simulink model "test_sim_model_scheduling_v1"  (R2023a)
settings: Solver=VariableStepAuto  StartTime=0.0  StopTime=10.0  RelTol=1e-3
values from neighbouring files (symbols this model uses):
  A = Amatrix(C1, C2, C3, Cf, Cs, Sx, Sy, x0(3), x0(4), w0(1), w0(2), u0(1), epsilon, g, lx, ly, mass, x0(6), x0(5), rho, u0(2), weight_part, wheel_rad)    [model_main_model_scheduling.m]
  A_inv = Amatrix(C1, C2, C3, Cf, Cs, Sx, Sy, x0(3), x0(4), w0_inv(1), w0_inv(2), u0(1), epsilon, g, lx, ly, mass, x0(6), x0(5), rho, u0(2), weight_part, wheel_rad)    [model_main_model_scheduling.m]
  B1 = B1matrix(C1, C2, C3, x0(3), x0(4), u0(1), epsilon, g, lx, mass, x0(6), x0(5), u0(2), weight_part, wheel_rad)    [model_main_model_scheduling.m]
  B1_inv = B1matrix(C1, C2, C3, x0(3), x0(4), u0(1), epsilon, g, lx, mass, x0(6), x0(5), u0(2), weight_part, wheel_rad)    [model_main_model_scheduling.m]
  B2 = B2matrix(Cf, Cs, Sx, Sy, x0(3), x0(4), w0(1), w0(2), epsilon, lx, ly, mass, x0(5), rho)    [model_main_model_scheduling.m]
  B2_inv = B2matrix(Cf, Cs, Sx, Sy, x0(3), x0(4), w0_inv(1), w0_inv(2), epsilon, lx, ly, mass, x0(5), rho)    [model_main_model_scheduling.m]
  C = Cmatrix    [model_main_model_scheduling.m]
  C_inv = Cmatrix    [model_main_model_scheduling.m]
  Ce = Cematrix    [model_main_model_scheduling.m]
  Ce_inv = Cematrix    [model_main_model_scheduling.m]
  D1 = D1matrix    [model_main_model_scheduling.m]
  D1_inv = D1matrix    [model_main_model_scheduling.m]
  D1e = D1ematrix    [model_main_model_scheduling.m]
  D1e_inv = D1ematrix    [model_main_model_scheduling.m]
  D2 = D2matrix    [model_main_model_scheduling.m]
  D2_inv = D2matrix    [model_main_model_scheduling.m]
  D2e = D2ematrix    [model_main_model_scheduling.m]
  D2e_inv = D2ematrix    [model_main_model_scheduling.m]
  e_init = y_init(2) - r_init(1)    [model_main_model_scheduling.m]
  K = Ke(:, 1:lenA)    [model_main_model_scheduling.m]
  K_inv = Ke_inv(:, 1:lenA)    [model_main_model_scheduling.m]
  KI = Ke(1, lenA+1:end)    [model_main_model_scheduling.m]
  KI_inv = Ke_inv(1, lenA+1:end)    [model_main_model_scheduling.m]
  x_init = [0 ... (first row only)    [model_main_model_scheduling.m]
libraries: simulink x6
settings Model: Creator=valer  LastModifiedBy=valer

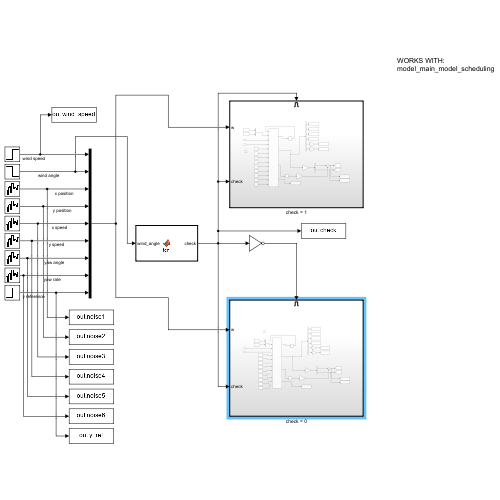
[thumbnail: Simulink's stored preview of the top-level diagram]
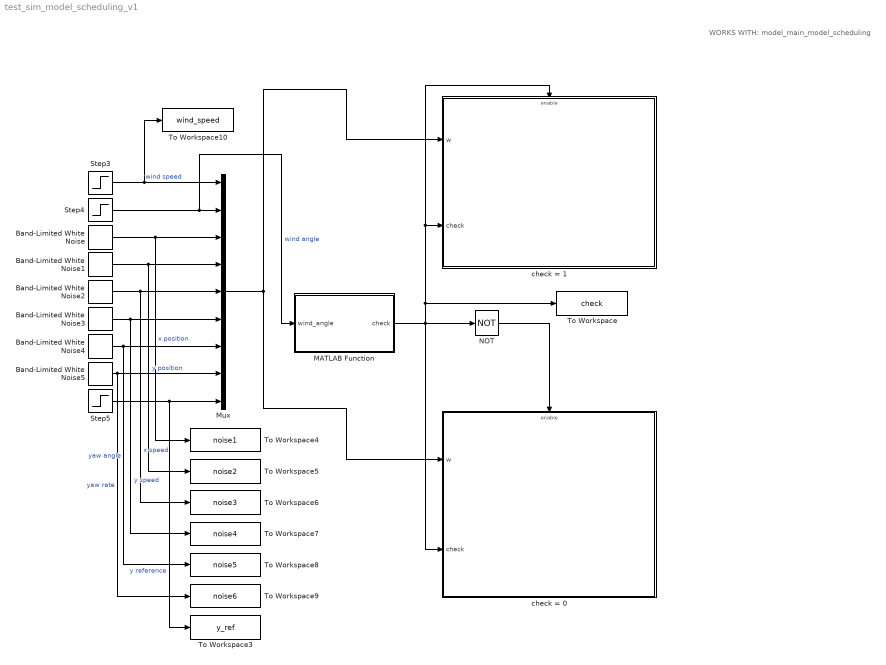
== system test_sim_model_scheduling_v1 ==
  note: WORKS WITH:
      | model_main_model_scheduling
  Band-Limited White Noise : simulink/Sources/Band-Limited White Noise  Cov=0.0001*0.01  Ts=0.05  seed=20000+10000*rand
  Band-Limited White Noise1 : simulink/Sources/Band-Limited White Noise  Cov=0.000285*0.01  Ts=0.05  seed=20000+10000*rand
  Band-Limited White Noise2 : simulink/Sources/Band-Limited White Noise  Cov=0.0009*0.01  Ts=0.05  seed=20000+10000*rand
  Band-Limited White Noise3 : simulink/Sources/Band-Limited White Noise  Cov=0.0009*0.01  Ts=0.05  seed=20000+10000*rand
  Band-Limited White Noise4 : simulink/Sources/Band-Limited White Noise  Cov=0.01 *pi/180*0.01  Ts=0.05  seed=20000+10000*rand
  Band-Limited White Noise5 : simulink/Sources/Band-Limited White Noise  Cov=0.54*pi/180*0.01  Ts=0.05  seed=20000+10000*rand
  MATLAB Function : MATLAB Function  TreatAsAtomicUnit=on
  Mux : Mux  Inputs=9
  NOT : Logic  Operator=NOT  IconShape=distinctive  AllPortsSameDT=off  OutDataTypeStr=boolean
  Step3 : Step  Time=5  After=25  SampleTime=0
  Step4 : Step  Time=0  After=-0.0001  SampleTime=0
  Step5 : Step  Time=5  After=0  SampleTime=0
  To Workspace : ToWorkspace  VariableName=check  SaveFormat=Timeseries  SampleTime=-1
  To Workspace10 : ToWorkspace  VariableName=wind_speed  SaveFormat=Timeseries  SampleTime=-1
  To Workspace3 : ToWorkspace  VariableName=y_ref  SaveFormat=Timeseries  SampleTime=-1
  To Workspace4 : ToWorkspace  VariableName=noise1  SaveFormat=Timeseries  SampleTime=-1
  To Workspace5 : ToWorkspace  VariableName=noise2  SaveFormat=Timeseries  SampleTime=-1
  To Workspace6 : ToWorkspace  VariableName=noise3  SaveFormat=Timeseries  SampleTime=-1
  To Workspace7 : ToWorkspace  VariableName=noise4  SaveFormat=Timeseries  SampleTime=-1
  To Workspace8 : ToWorkspace  VariableName=noise5  SaveFormat=Timeseries  SampleTime=-1
  To Workspace9 : ToWorkspace  VariableName=noise6  SaveFormat=Timeseries  SampleTime=-1
  check = 0 : Subsystem
  check = 1 : Subsystem
  wires:
  Step3/1 -> Mux/1, To Workspace10/1  "wind speed"
  Band-Limited White Noise4/1 -> To Workspace8/1, Mux/7  "yaw angle"
  Step5/1 -> To Workspace3/1, Mux/9  "y reference"
  Band-Limited White Noise3/1 -> To Workspace7/1, Mux/6  "y speed"
  Band-Limited White Noise2/1 -> To Workspace6/1, Mux/5  "x speed"
  Band-Limited White Noise5/1 -> To Workspace9/1, Mux/8  "yaw rate"
  Band-Limited White Noise/1 -> To Workspace4/1, Mux/3  "x position"
  Band-Limited White Noise1/1 -> To Workspace5/1, Mux/4  "y position"
  Step4/1 -> MATLAB Function/1(wind_angle), Mux/2  "wind angle"
  Mux/1 -> check = 1/1(w), check = 0/1(w)
  MATLAB Function/1(check) -> NOT/1, To Workspace/1, check = 1/Enable, check = 1/2(check), check = 0/2(check)
  NOT/1 -> check = 0/Enable

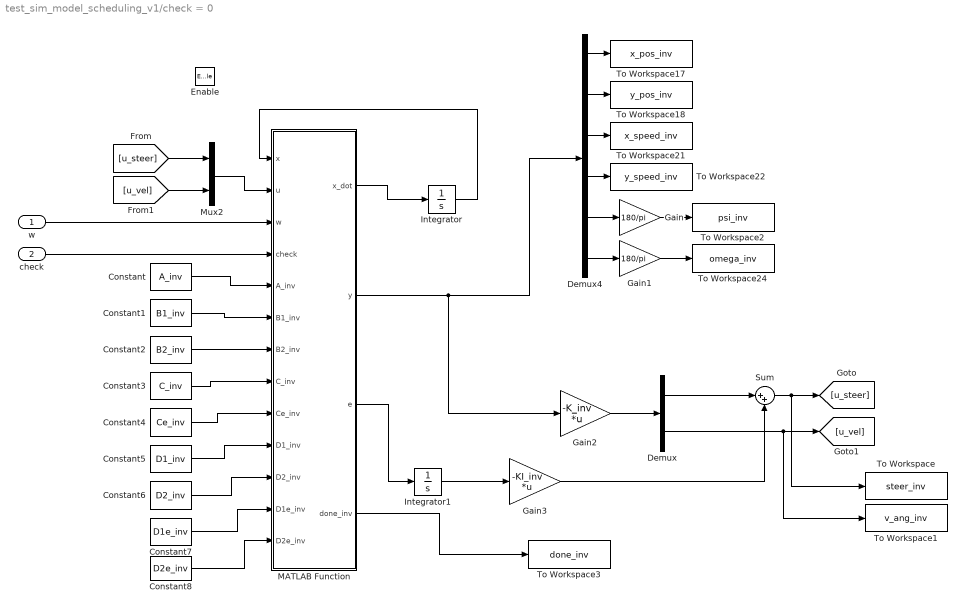
== system test_sim_model_scheduling_v1/check = 0 ==
  w : Inport
  check : Inport  Port=2
  Enable : EnablePort
  Constant : Constant  Value=A_inv
  Constant1 : Constant  Value=B1_inv
  Constant2 : Constant  Value=B2_inv
  Constant3 : Constant  Value=C_inv
  Constant4 : Constant  Value=Ce_inv
  Constant5 : Constant  Value=D1_inv
  Constant6 : Constant  Value=D2_inv
  Constant7 : Constant  Value=D1e_inv
  Constant8 : Constant  Value=D2e_inv
  Demux : Demux  Outputs=2
  Demux4 : Demux  Outputs=6
  Gain : Gain  Gain=180/pi
  Gain1 : Gain  Gain=180/pi
  Gain2 : Gain  Gain=-K_inv  Multiplication=Matrix(K*u)
  Gain3 : Gain  Gain=-KI_inv  Multiplication=Matrix(K*u)
  Integrator : Integrator  InitialCondition=x_init
  Integrator1 : Integrator  InitialCondition=e_init
  MATLAB Function : MATLAB Function  TreatAsAtomicUnit=on
  Mux2 : Mux  Inputs=2
  Sum : Sum  Inputs=|++
  To Workspace : ToWorkspace  VariableName=steer_inv  SaveFormat=Timeseries  SampleTime=-1
  To Workspace1 : ToWorkspace  VariableName=v_ang_inv  SaveFormat=Timeseries  SampleTime=-1
  To Workspace17 : ToWorkspace  VariableName=x_pos_inv  SaveFormat=Timeseries  SampleTime=-1
  To Workspace18 : ToWorkspace  VariableName=y_pos_inv  SaveFormat=Timeseries  SampleTime=-1
  To Workspace2 : ToWorkspace  VariableName=psi_inv  SaveFormat=Timeseries  SampleTime=-1
  To Workspace21 : ToWorkspace  VariableName=x_speed_inv  SaveFormat=Timeseries  SampleTime=-1
  To Workspace22 : ToWorkspace  VariableName=y_speed_inv  SaveFormat=Timeseries  SampleTime=-1
  To Workspace24 : ToWorkspace  VariableName=omega_inv  SaveFormat=Timeseries  SampleTime=-1
  To Workspace3 : ToWorkspace  VariableName=done_inv  SaveFormat=Timeseries  SampleTime=-1
  wires:
  w/1 -> MATLAB Function/3(w)
  MATLAB Function/1(x_dot) -> Integrator/1
  Demux4/6 -> Gain1/1
  Demux4/4 -> To Workspace22/1
  Constant2/1 -> MATLAB Function/7(B2_inv)
  MATLAB Function/3(e) -> Integrator1/1
  Gain1/1 -> To Workspace24/1
  Constant1/1 -> MATLAB Function/6(B1_inv)
  Constant4/1 -> MATLAB Function/9(Ce_inv)
  Gain2/1 -> Demux/1
  Demux/1 -> Sum/1
  Integrator1/1 -> Gain3/1
  [u_vel] -> Mux2/2
  Demux4/3 -> To Workspace21/1
  Constant3/1 -> MATLAB Function/8(C_inv)
  [u_steer] -> Mux2/1
  Demux4/2 -> To Workspace18/1
  Sum/1 -> To Workspace/1, [u_steer]
  Constant/1 -> MATLAB Function/5(A_inv)
  Gain/1 -> To Workspace2/1
  Constant6/1 -> MATLAB Function/11(D2_inv)
  Constant7/1 -> MATLAB Function/12(D1e_inv)
  Constant8/1 -> MATLAB Function/13(D2e_inv)
  Mux2/1 -> MATLAB Function/2(u)
  Demux4/1 -> To Workspace17/1
  MATLAB Function/2(y) -> Gain2/1, Demux4/1
  Constant5/1 -> MATLAB Function/10(D1_inv)
  Integrator/1 -> MATLAB Function/1(x)
  Demux4/5 -> Gain/1
  Demux/2 -> [u_vel], To Workspace1/1
  check/1 -> MATLAB Function/4(check)
  MATLAB Function/4(done_inv) -> To Workspace3/1
  Gain3/1 -> Sum/2

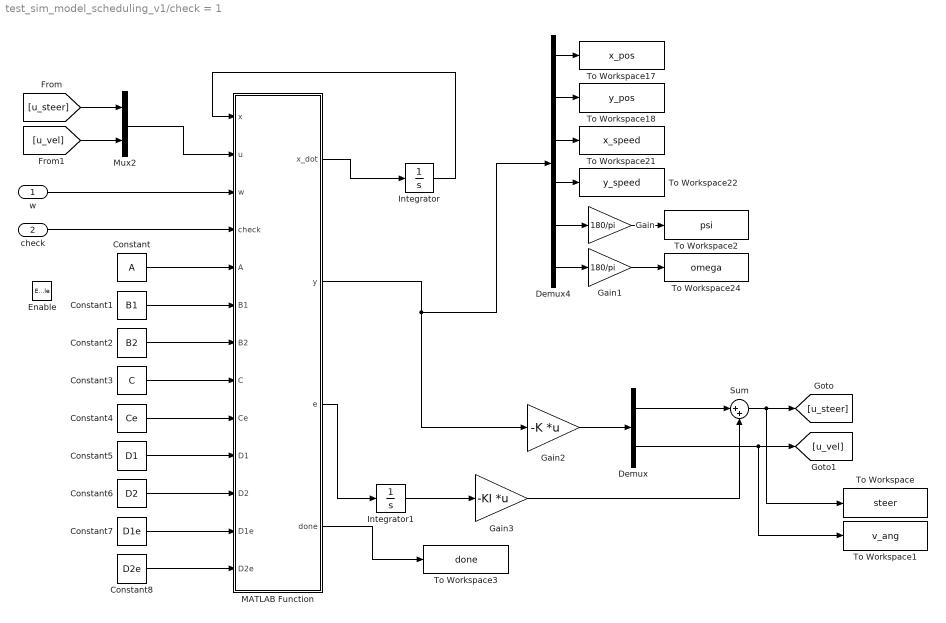
== system test_sim_model_scheduling_v1/check = 1 ==
  w : Inport
  check : Inport  Port=2
  Enable : EnablePort
  Constant : Constant  Value=A
  Constant1 : Constant  Value=B1
  Constant2 : Constant  Value=B2
  Constant3 : Constant  Value=C
  Constant4 : Constant  Value=Ce
  Constant5 : Constant  Value=D1
  Constant6 : Constant  Value=D2
  Constant7 : Constant  Value=D1e
  Constant8 : Constant  Value=D2e
  Demux : Demux  Outputs=2
  Demux4 : Demux  Outputs=6
  Gain : Gain  Gain=180/pi
  Gain1 : Gain  Gain=180/pi
  Gain2 : Gain  Gain=-K  Multiplication=Matrix(K*u)
  Gain3 : Gain  Gain=-KI  Multiplication=Matrix(K*u)
  Integrator : Integrator  InitialCondition=x_init
  Integrator1 : Integrator  InitialCondition=e_init
  MATLAB Function : MATLAB Function  TreatAsAtomicUnit=on
  Mux2 : Mux  Inputs=2
  Sum : Sum  Inputs=|++
  To Workspace : ToWorkspace  VariableName=steer  SaveFormat=Timeseries  SampleTime=-1
  To Workspace1 : ToWorkspace  VariableName=v_ang  SaveFormat=Timeseries  SampleTime=-1
  To Workspace17 : ToWorkspace  VariableName=x_pos  SaveFormat=Timeseries  SampleTime=-1
  To Workspace18 : ToWorkspace  VariableName=y_pos  SaveFormat=Timeseries  SampleTime=-1
  To Workspace2 : ToWorkspace  VariableName=psi  SaveFormat=Timeseries  SampleTime=-1
  To Workspace21 : ToWorkspace  VariableName=x_speed  SaveFormat=Timeseries  SampleTime=-1
  To Workspace22 : ToWorkspace  VariableName=y_speed  SaveFormat=Timeseries  SampleTime=-1
  To Workspace24 : ToWorkspace  VariableName=omega  SaveFormat=Timeseries  SampleTime=-1
  To Workspace3 : ToWorkspace  VariableName=done  SaveFormat=Timeseries  SampleTime=-1
  wires:
  Demux/2 -> To Workspace1/1, [u_vel]
  Demux4/5 -> Gain/1
  Integrator/1 -> MATLAB Function/1(x)
  Constant5/1 -> MATLAB Function/10(D1)
  MATLAB Function/2(y) -> Gain2/1, Demux4/1
  Demux4/1 -> To Workspace17/1
  Gain3/1 -> Sum/2
  Mux2/1 -> MATLAB Function/2(u)
  Constant8/1 -> MATLAB Function/13(D2e)
  Constant7/1 -> MATLAB Function/12(D1e)
  Constant6/1 -> MATLAB Function/11(D2)
  Gain/1 -> To Workspace2/1
  Constant/1 -> MATLAB Function/5(A)
  Sum/1 -> [u_steer], To Workspace/1
  Demux4/2 -> To Workspace18/1
  [u_steer] -> Mux2/1
  Constant3/1 -> MATLAB Function/8(C)
  Demux4/3 -> To Workspace21/1
  [u_vel] -> Mux2/2
  Integrator1/1 -> Gain3/1
  Demux/1 -> Sum/1
  Gain2/1 -> Demux/1
  Constant4/1 -> MATLAB Function/9(Ce)
  Constant1/1 -> MATLAB Function/6(B1)
  Gain1/1 -> To Workspace24/1
  MATLAB Function/3(e) -> Integrator1/1
  Constant2/1 -> MATLAB Function/7(B2)
  Demux4/4 -> To Workspace22/1
  Demux4/6 -> Gain1/1
  MATLAB Function/1(x_dot) -> Integrator/1
  w/1 -> MATLAB Function/3(w)
  check/1 -> MATLAB Function/4(check)
  MATLAB Function/4(done) -> To Workspace3/1

== matlab function test_sim_model_scheduling_v1/check = 0/MATLAB Function ==
  data: x input; x_dot output; u input; y output; w input; check input; e output; A_inv input; B1_inv input; B2_inv input; C_inv input; Ce_inv input; D1_inv input; D2_inv input; D1e_inv input; D2e_inv input; done_inv output
function [x_dot, y, e,done_inv] = fcn(x,u,w,check, A_inv,B1_inv,B2_inv,C_inv,Ce_inv,D1_inv,D2_inv,D1e_inv,D2e_inv)

x_dot = [0;0;0;0;0;0];
y = [0;0;0;0;0;0];
e = 0;
done_inv = 0;
if check == 0
    done_inv = 1;
    % linear system
    x_dot = A_inv * x + B1_inv * u + B2_inv * w;
    y = C_inv * x + D1_inv * u + D2_inv * w;
    e = Ce_inv' * x + D1e_inv' * u + D2e_inv' * w;
end

== matlab function test_sim_model_scheduling_v1/check = 1/MATLAB Function ==
  data: x input; x_dot output; u input; y output; w input; check input; e output; A input; B1 input; B2 input; C input; Ce input; D1 input; D2 input; D1e input; D2e input; done output
function [x_dot, y, e, done] = fcn(x,u,w,check, A,B1,B2,C,Ce,D1,D2,D1e,D2e)
x_dot = [0;0;0;0;0;0];
y = [0;0;0;0;0;0];
e = 0;
done = 0;
if check ~= 0
    done = 1;
    % linear system
    x_dot = A * x + B1 * u + B2 * w;
    y = C * x + D1 * u + D2 * w;
    e = Ce' * x + D1e' * u + D2e' * w;
end

== matlab function test_sim_model_scheduling_v1/MATLAB Function ==
  data: wind_angle input; check output
function check = fcn(wind_angle)
check = 1;

if wind_angle >= 0
    check = 1;
elseif wind_angle < 0 
    check = 0;
end
